simulink model "Inter_story_damped_structure_MFD_reference"  (R2024a)
settings: Solver=ode4  StartTime=0.0  StopTime=tend  FixedStep=dt  RelTol=1e-3
values from neighbouring files (symbols this model uses):
  A0 = 0.4    [Base_isolated_structure_main.m]    (also in Inter_story_damped_structure_MBW_main.m = [zeros(Ns) eye(Ns);-M\K -M\C]; Inter_story_damped_structure_MFD_main.m = [zeros(Ns) eye(Ns);-M\K -M\C])
  B1 = [zeros(Ns,1+Ns);-ones(Ns,1) -M\Re]    [Inter_story_damped_structure_MBW_main.m]    (also in Inter_story_damped_structure_MFD_main.m)
  C0 = eye(2*Ns)    [Inter_story_damped_structure_MBW_main.m]    (also in Inter_story_damped_structure_MFD_main.m)
  coe = [A,gamma,beta,n]    [BLWN_training_data_prep.m]    (also in Base_isolated_structure_main.m = [-a_0*dta,dta,b_0-a_0*b_1,b_1,UL]; Inter_story_damped_structure_MFD_main.m = [-a_0*dta,dta,b_0-a_0*b_1,b_1,UL])
  D1 = zeros(2*Ns,1+Ns)    [Inter_story_damped_structure_MBW_main.m]    (also in Inter_story_damped_structure_MFD_main.m)
  dt = 0.002    [BLWN_training_data_prep.m]    (also in Base_isolated_structure_main.m; Inter_story_damped_structure_MBW_main.m; Inter_story_damped_structure_MFD_main.m)
  GL = zeros(lim-1,1);GL(1)=-alpha    [Base_isolated_structure_main.m]    (also in Inter_story_damped_structure_MFD_main.m)
  k0 = 0.5e-3    (= 0.0005)    [BLWN_training_data_prep.m]    (also in Base_isolated_structure_main.m = 500000; Inter_story_damped_structure_MFD_main.m)
  Ns = 5    [Inter_story_damped_structure_MBW_main.m]    (also in Inter_story_damped_structure_MFD_main.m)
  UL = i-1    [Base_isolated_structure_main.m]    (also in Inter_story_damped_structure_MFD_main.m)
settings Model: Creator=hongwei  LastModifiedBy=li292
settings DataIOCC: SaveTime=off  ReturnWorkspaceOutputs=off
settings OptimizationCC: ReuseModelBlockBuffer=off
settings RTWCC: GPUComputeCapability=3.5

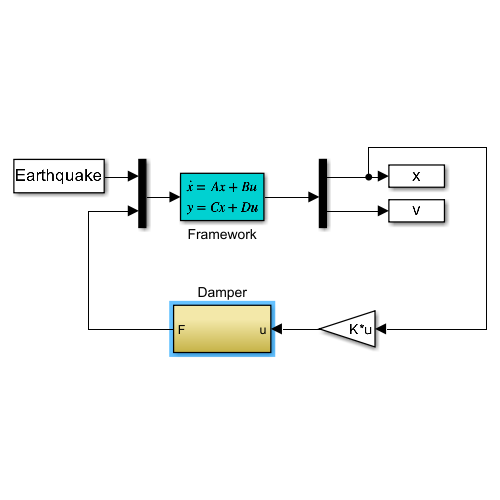
[thumbnail: Simulink's stored preview of the top-level diagram]
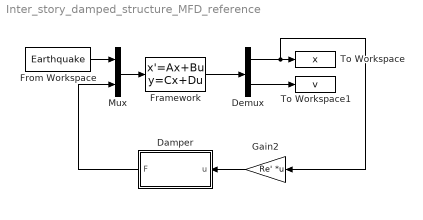
== system Inter_story_damped_structure_MFD_reference ==
  Damper : Subsystem
  Demux : Demux  Outputs=2
  Framework : StateSpace  A=A0  B=B1  C=C0  D=D1  InitialCondition=zeros(2*Ns,1)
  From Workspace : FromWorkspace  VariableName=Earthquake  SampleTime=dt
  Gain2 : Gain  Gain=Re'  Multiplication=Matrix(K*u)
  Mux : Mux  Inputs=2
  To Workspace : ToWorkspace  VariableName=x  SampleTime=-1
  To Workspace1 : ToWorkspace  VariableName=v  SampleTime=-1
  wires:
  Framework/1 -> Demux/1
  Demux/1 -> To Workspace/1, Gain2/1
  Demux/2 -> To Workspace1/1
  Mux/1 -> Framework/1
  From Workspace/1 -> Mux/1
  Damper/1(F) -> Mux/2
  Gain2/1 -> Damper/1(u)

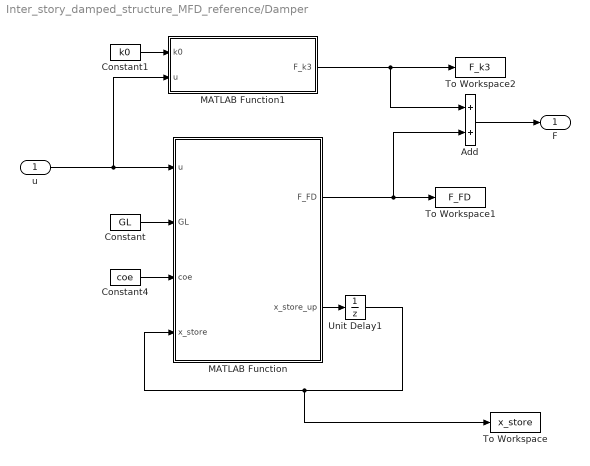
== system Inter_story_damped_structure_MFD_reference/Damper ==
  u : Inport
  Add : Sum
  Constant : Constant  Value=GL  VectorParams1D=off
  Constant1 : Constant  Value=k0  VectorParams1D=off
  Constant4 : Constant  Value=coe  VectorParams1D=off
  MATLAB Function : MATLAB Function  TreatAsAtomicUnit=on
  MATLAB Function1 : MATLAB Function  TreatAsAtomicUnit=on
  To Workspace : ToWorkspace  VariableName=x_store  SampleTime=-1
  To Workspace1 : ToWorkspace  VariableName=F_FD  SampleTime=-1
  To Workspace2 : ToWorkspace  VariableName=F_k3  SampleTime=-1
  Unit Delay1 : UnitDelay  InitialCondition=[zeros(Ns,UL)]  SampleTime=-1  HasFrameUpgradeWarning=on
  F : Outport  VectorParamsAs1DForOutWhenUnconnected=off
  wires:
  u/1 -> MATLAB Function1/2(u), MATLAB Function/1(u)
  Constant4/1 -> MATLAB Function/3(coe)
  MATLAB Function/2(x_store_up) -> Unit Delay1/1
  MATLAB Function/1(F_FD) -> To Workspace1/1, Add/2
  Unit Delay1/1 -> To Workspace/1, MATLAB Function/4(x_store)
  Constant/1 -> MATLAB Function/2(GL)
  Constant1/1 -> MATLAB Function1/1(k0)
  MATLAB Function1/1(F_k3) -> To Workspace2/1, Add/1
  Add/1 -> F/1

== matlab function Inter_story_damped_structure_MFD_reference/Damper/MATLAB Function1 ==
  data: k0 input; F_k3 output; u input
function F_k3  = fcn(k0,u)
F_k3=k0*u.^3;

== matlab function Inter_story_damped_structure_MFD_reference/Damper/MATLAB Function ==
  data: F_FD output; u input; GL input; coe input; x_store input; x_store_up output
function [F_FD,x_store_up] = fcn(u,GL,coe,x_store)
A=coe(1); B=coe(2); C=coe(3); D=coe(4); UL=coe(5);


F_FD = C*x_store(:,1)+D*u;
x_store_up=x_store;
x_store_up(:,2:UL)=x_store(:,1:UL-1);
x_store_up(:,1)=A*x_store(:,1)+B*u-x_store*GL(1:UL);
